simulink model "PMSM_Model_fixed"  (R2022b)
settings: Solver=ode23t  StartTime=0.0  StopTime=0.5  RelTol=1e-3
model workspace (MAT data in the model file):
  Ki = 1000
  Kp = 2
  Ts_ctrl = 0.0001
  Ts_norm = 1
  Vdc = 100
  fsw = 10000
  p = 6
undefined symbols (not defined in the file): docblock
libraries: nesl_utility x11, fl_lib x10, ee_lib x4, spsTriangleGeneratorLib x1
settings Model: Creator=59263  LastModifiedBy=59263

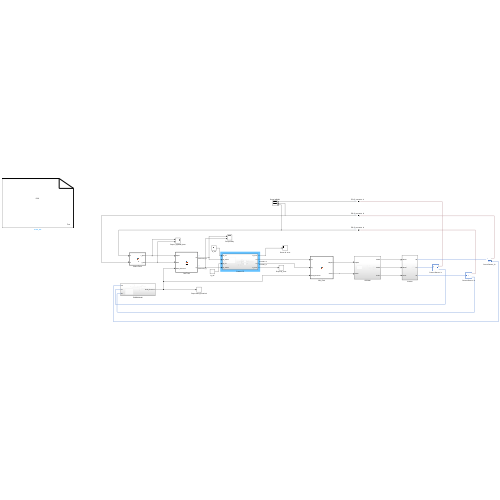
[thumbnail: Simulink's stored preview of the top-level diagram]
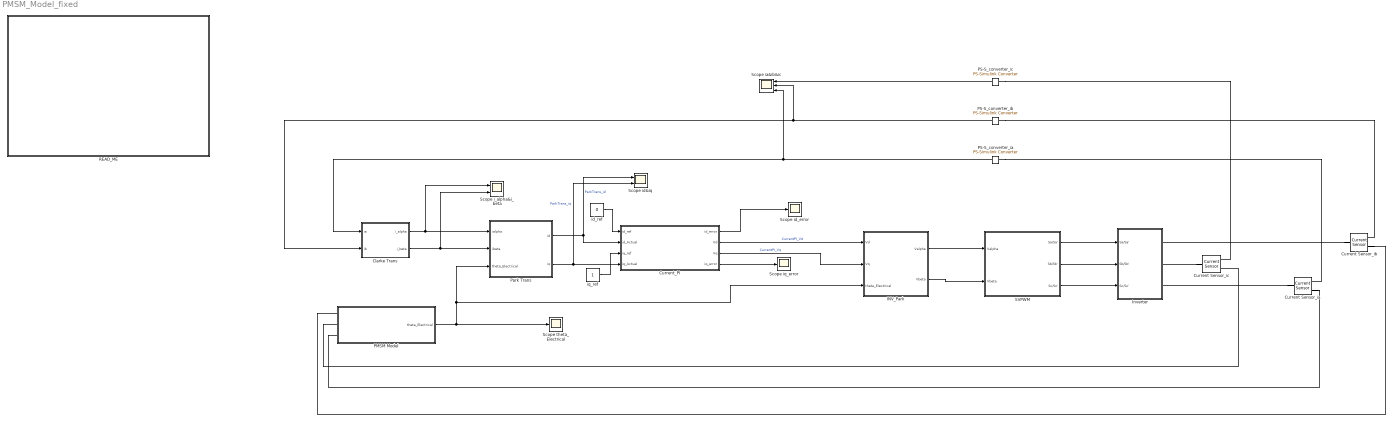
== system PMSM_Model_fixed ==
  Clarke Trans : MATLAB Function  TreatAsAtomicUnit=on
  Current Sensor_ia : fl_lib/Electrical/Electrical Sensors/Current Sensor
  Current Sensor_ib : fl_lib/Electrical/Electrical Sensors/Current Sensor
  Current Sensor_ic : fl_lib/Electrical/Electrical Sensors/Current Sensor
  Current_PI : Subsystem
  INV_Park : MATLAB Function  TreatAsAtomicUnit=on
  Inverter : Subsystem
  PMSM Model : Subsystem
  PS-S_converter_ia : nesl_utility/PS-Simulink Converter  PhysicalDomain=network_engine_domain  SubClassName=ps_output  LeftPortType=input  RightPortType=output  PseudoPeriodic=off  Frequencies=[]  VectorFormat=inherit  Unit=A  AffineConversion=off
  PS-S_converter_ib : nesl_utility/PS-Simulink Converter  PhysicalDomain=network_engine_domain  SubClassName=ps_output  LeftPortType=input  RightPortType=output  PseudoPeriodic=off  Frequencies=[]  VectorFormat=inherit  Unit=A  AffineConversion=off
  PS-S_converter_ic : nesl_utility/PS-Simulink Converter  PhysicalDomain=network_engine_domain  SubClassName=ps_output  LeftPortType=input  RightPortType=output  PseudoPeriodic=off  Frequencies=[]  VectorFormat=inherit  Unit=inherit  AffineConversion=off
  Park Trans : MATLAB Function  TreatAsAtomicUnit=on
  READ_ME : Subsystem  InitFcn=docblock('save_document',gcb);  mask(DocBlock){ECoderFlag=, DocumentType=Text}
      mask prompts: ECoderFlag "Simulink:masks:DocBlockEmbeddedCoderFlagLabel_MP"; DocumentType "Simulink:masks:DocBlockDocTypeLabel_MP"
      mask help:
      | PMSM 矢量控制（FOC）仿真模型 —— 表贴式 PMSM，i_d* = 0，i_q* = 1 A
      |
      | 【功能分层】
      |   Inverter     三相两电平电压源逆变器（3 x Half-Bridge）+ 直流母线 + 电压传感
      |   PMSM Model   PMSM 本体 + 旋转传感器 + 位置处理，输出电角度 theta_Electrical
      |   Current_PI   dq 电流环（离散 PI + 一拍计算延迟），输出 Vd / Vq 及 id/iq 误差
      |   SVPWM        空间矢量调制：abc_PWM（扇区/T1T2/占空比）+ 载波比较 + 互补门极
      |
      | 【模型工作区变量】改参数请改这里，不要钻进子系统改
      |   Kp      = 2      电流环比例增益
      |   Ki      = 1000   电流环积分增益（Ki/Kp = R/L = 500，Kp = wc*L）
      |   Vdc     = 100    直流母线电压 [V]（同时驱动 DC 源、SVPWM 的 Vdc）
      |   Ts_norm = 1      SVPWM 归一化周期（Ts=1 时 Da/Db/Dc 直接就是占空比）
      |   Ts_ctrl = 1e-4   电流环采样周期 [s]，10 kHz，与载波同频
      |   fsw     = 1e4    三角载波频率 [Hz]
      |   p       = 6      极对数（同时驱动 PMSM 本体和 theta 换算的 Gain）
      |
      | 【运行】StopTime = 0.5 s，变步长 ode23t，RelTol = 1e-3
      |
      | 【改参数时的联动关系】
      |   Vdc  ->  同时影响 DC 源、SVPWM 占空比计算
      |         ->  PI 脚本里硬编码的限幅 limit = 57 V (= Vdc/sqrt(3)) 也要同步改
      |   Ts_ctrl/p/fsw -> 见 Current_PI 与 SVPWM 子系统里的说明
      settings: DeleteFcn=docblock('close_document',gcb);  PreSaveFcn=docblock('save_document',gcb);  OpenFcn=docblock('edit_document',gcb);
      settings: LibrarySourceBlock=|
      | simulink/Model-Wide
      | Utilities/DocBlock
      mask TypeOptions DocumentType: Simulink:masks:Text | Simulink:masks:RTF | Simulink:masks:HTML
      mask Display:
      | plot([.8 0 0 1 1 .8 .8 1],[1 1 0 0 .8 1 .8 .8]);
      | text(.5,.6,'DOC','horizontalalignment','center');
      | text(.95,.05,get_param(gcb,'DocumentType'),'verticalalignment','bottom','horizontalalignment','right');
  SVPWM : Subsystem
  Scope i_alpha&i_beta : Scope  NumInputPorts=2
  Scope ia&ib&ic : Scope  NumInputPorts=3
  Scope id&iq : Scope  NumInputPorts=2
  Scope id_error : Scope
  Scope iq_error : Scope
  Scope theta_Electrical : Scope
  id_ref : Constant  Value=0
  iq_ref : Constant
  wires:
  PS-S_converter_ia/1 -> Clarke Trans/1(ia), Scope ia&ib&ic/3
  PS-S_converter_ib/1 -> Clarke Trans/2(ib), Scope ia&ib&ic/2
  Clarke Trans/1(i_alpha) -> Scope i_alpha&i_beta/1, Park Trans/1(ialpha)
  Clarke Trans/2(i_beta) -> Scope i_alpha&i_beta/2, Park Trans/2(ibeta)
  Park Trans/1(id) -> Current_PI/2(id_Actual), Scope id&iq/1  "ParkTrans_id"
  Park Trans/2(iq) -> Current_PI/4(iq_Actual), Scope id&iq/2  "ParkTrans_iq"
  INV_Park/1(Valpha) -> SVPWM/1(Valpha)
  INV_Park/2(Vbeta) -> SVPWM/2(Vbeta)
  SVPWM/1(Sa/Sa') -> Inverter/1(Sa/Sa')
  SVPWM/2(Sb/Sb') -> Inverter/2(Sb/Sb')
  SVPWM/3(Sc/Sc') -> Inverter/3(Sc/Sc')
  Current_PI/1(id_error) -> Scope id_error/1
  Current_PI/2(Vd) -> INV_Park/1(Vd)  "CurrentPI_Vd"
  Current_PI/3(Vq) -> INV_Park/2(Vq)  "CurrentPI_Vq"
  Current_PI/4(iq_error) -> Scope iq_error/1
  PMSM Model/1(theta_Electrical) -> Scope theta_Electrical/1, Park Trans/3(theta_Electrical), INV_Park/3(theta_Electrical)
  PS-S_converter_ic/1 -> Scope ia&ib&ic/1
  id_ref/1 -> Current_PI/1(id_ref)
  iq_ref/1 -> Current_PI/3(iq_ref)
  connections:
  PS-S_converter_ia/LConn1 -- Current Sensor_ia/RConn1
  PS-S_converter_ib/LConn1 -- Current Sensor_ib/RConn1
  PS-S_converter_ic/LConn1 -- Current Sensor_ic/RConn1
  Current Sensor_ib/LConn1 -- Inverter/RConn1
  Current Sensor_ic/LConn1 -- Inverter/RConn2
  Current Sensor_ia/LConn1 -- Inverter/RConn3
  Current Sensor_ib/RConn2 -- PMSM Model/LConn1
  PMSM Model/LConn2 -- Current Sensor_ic/RConn2
  Current Sensor_ia/RConn2 -- PMSM Model/LConn3

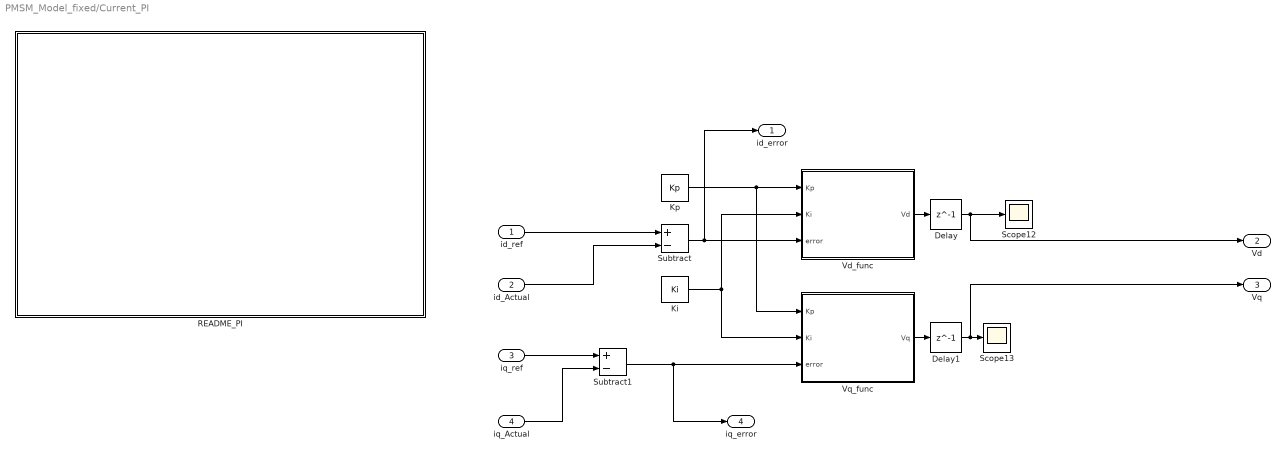
== system PMSM_Model_fixed/Current_PI ==
  id_ref : Inport
  id_Actual : Inport  Port=2
  iq_ref : Inport  Port=3
  iq_Actual : Inport  Port=4
  Delay : Delay  DelayLength=1  SampleTime=Ts_ctrl
  Delay1 : Delay  DelayLength=1  SampleTime=Ts_ctrl
  Ki : Constant  Value=Ki
  Kp : Constant  Value=Kp
  README_PI : Subsystem  InitFcn=docblock('save_document',gcb);  mask(DocBlock){ECoderFlag=, DocumentType=Text}
      mask prompts: ECoderFlag "Simulink:masks:DocBlockEmbeddedCoderFlagLabel_MP"; DocumentType "Simulink:masks:DocBlockDocTypeLabel_MP"
      mask help:
      | dq 轴电流环（离散 PI）
      |
      | 【接口】
      |   输入：id_ref、id_Actual、iq_ref、iq_Actual
      |   输出：id_error、Vd、Vq、iq_error
      |
      | 【结构】
      |   Subtract(+-)  -> id_error -> Vd_func -> Delay (Ts_ctrl) -> Vd
      |   Subtract1(+-) -> iq_error -> Vq_func -> Delay1(Ts_ctrl) -> Vq
      |
      | 【增益】Kp / Ki 引用模型工作区变量（默认 2 / 1000）
      |   整定依据：对象 1/(Ls+R)，L = 1 mH，R = 0.5 ohm
      |     零极点对消：Ki/Kp = R/L = 500
      |     穿越频率  ：wc = Kp/L = 2000 rad/s ≈ 318 Hz（约 fsw/31）
      |     相位裕度  ：PM ≈ 90 - wc*Td ≈ 67 度（Td ≈ 2 个采样周期）
      |
      | 【!! 采样时间一致性 !!】
      |   两个 PI 图表必须保持 ChartUpdate = DISCRETE、SampleTime = 1e-4，
      |   并且脚本里的字面量 Ts 必须等于该采样时间。
      |   若图表是 INHERITED（连续），在变步长求解器下积分量会被重复累加
      |   约两个数量级，整定参数完全失效 —— 这是最难查的一类静默错误。
      |
      | 【限幅】Vd / Vq 的限幅 ±57 V 硬编码在脚本里 = Vdc/sqrt(3)，改 Vdc 时要同步改。
      settings: DeleteFcn=docblock('close_document',gcb);  PreSaveFcn=docblock('save_document',gcb);  OpenFcn=docblock('edit_document',gcb);
      settings: LibrarySourceBlock=|
      | simulink/Model-Wide
      | Utilities/DocBlock
      mask TypeOptions DocumentType: Simulink:masks:Text | Simulink:masks:RTF | Simulink:masks:HTML
      mask Display:
      | plot([.8 0 0 1 1 .8 .8 1],[1 1 0 0 .8 1 .8 .8]);
      | text(.5,.6,'DOC','horizontalalignment','center');
      | text(.95,.05,get_param(gcb,'DocumentType'),'verticalalignment','bottom','horizontalalignment','right');
  Scope12 : Scope
  Scope13 : Scope
  Subtract : Sum  Inputs=+-
  Subtract1 : Sum  Inputs=+-
  Vd_func : MATLAB Function  TreatAsAtomicUnit=on
  Vq_func : MATLAB Function  TreatAsAtomicUnit=on
  id_error : Outport
  Vd : Outport  Port=2
  Vq : Outport  Port=3
  iq_error : Outport  Port=4
  wires:
  Vd_func/1(Vd) -> Delay/1
  Delay/1 -> Vd/1, Scope12/1
  Subtract/1 -> id_error/1, Vd_func/3(error)
  Vq_func/1(Vq) -> Delay1/1
  id_ref/1 -> Subtract/1
  Delay1/1 -> Vq/1, Scope13/1
  Ki/1 -> Vq_func/2(Ki), Vd_func/2(Ki)
  Subtract1/1 -> Vq_func/3(error), iq_error/1
  id_Actual/1 -> Subtract/2
  Kp/1 -> Vd_func/1(Kp), Vq_func/1(Kp)
  iq_ref/1 -> Subtract1/1
  iq_Actual/1 -> Subtract1/2

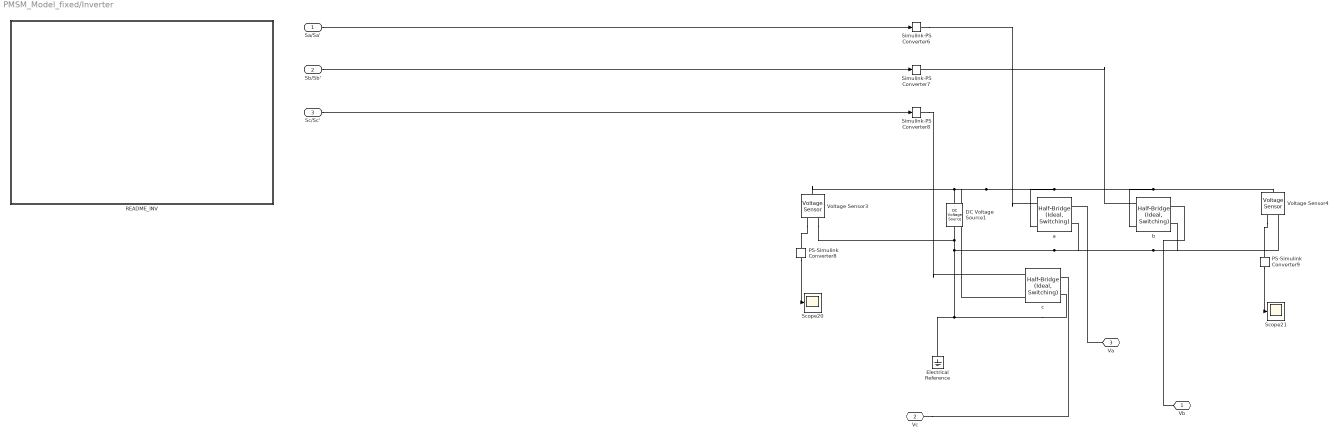
== system PMSM_Model_fixed/Inverter ==
  Sa/Sa' : Inport
  Sb/Sb' : Inport  Port=2
  Sc/Sc' : Inport  Port=3
  DC Voltage Source1 : fl_lib/Electrical/Electrical Sources/DC Voltage Source  v0=Vdc V
  Electrical Reference : fl_lib/Electrical/Electrical Elements/Electrical Reference
  PS-Simulink Converter8 : nesl_utility/PS-Simulink Converter  PhysicalDomain=network_engine_domain  SubClassName=ps_output  LeftPortType=input  RightPortType=output  PseudoPeriodic=off  Frequencies=[]  VectorFormat=inherit  Unit=inherit  AffineConversion=off
  PS-Simulink Converter9 : nesl_utility/PS-Simulink Converter  PhysicalDomain=network_engine_domain  SubClassName=ps_output  LeftPortType=input  RightPortType=output  PseudoPeriodic=off  Frequencies=[]  VectorFormat=inherit  Unit=inherit  AffineConversion=off
  README_INV : Subsystem  InitFcn=docblock('save_document',gcb);  mask(DocBlock){ECoderFlag=, DocumentType=Text}
      mask prompts: ECoderFlag "Simulink:masks:DocBlockEmbeddedCoderFlagLabel_MP"; DocumentType "Simulink:masks:DocBlockDocTypeLabel_MP"
      mask help:
      | 三相两电平电压源型逆变器
      |
      | 【接口】
      |   信号输入 Sa/Sa'、Sb/Sb'、Sc/Sc'：每路 2 元素向量 [上管门极, 下管门极]，互补
      |   物理端口 Va / Vb / Vc（块上顺序是 Vb / Vc / Va）：三个桥臂中点
      |
      | 【器件设置】
      |   device_type = MOSFET (Ideal, Switching)，mosfet_Vth = 0.5 V
      |   ! 阈值必须匹配门极信号电平（0/1 逻辑 -> 0.5 V）。
      |     若换成 GTO，阈值变成 gto_Vgt = 6 V，0/1 信号将无法开通。
      |   ! diode_param = include.no：半桥不含反并联续流二极管，
      |     因此必须用互补门极提供续流通路（已由 SVPWM 侧的 NOT + Mux 保证）。
      |     真实逆变器一定有体二极管或反并联二极管。
      |
      | 【其他】
      |   DC Voltage Source1 的 v0 = Vdc（模型工作区变量）
      |   Voltage Sensor3/4 跨接在直流母线上，测的是母线电压（冗余，控制未使用）
      settings: DeleteFcn=docblock('close_document',gcb);  PreSaveFcn=docblock('save_document',gcb);  OpenFcn=docblock('edit_document',gcb);
      settings: LibrarySourceBlock=|
      | simulink/Model-Wide
      | Utilities/DocBlock
      mask TypeOptions DocumentType: Simulink:masks:Text | Simulink:masks:RTF | Simulink:masks:HTML
      mask Display:
      | plot([.8 0 0 1 1 .8 .8 1],[1 1 0 0 .8 1 .8 .8]);
      | text(.5,.6,'DOC','horizontalalignment','center');
      | text(.95,.05,get_param(gcb,'DocumentType'),'verticalalignment','bottom','horizontalalignment','right');
  Scope20 : Scope
  Scope21 : Scope
  Simulink-PS Converter6 : nesl_utility/Simulink-PS Converter  PhysicalDomain=network_engine_domain  SubClassName=ps_input  LeftPortType=input  RightPortType=output  PseudoPeriodic=off  Frequencies=[]  NoiseDistribution=none  NoiseParameters=[]  Unit=1  AffineConversion=off  FilteringAndDerivatives=provide  SimscapeFilterOrder=1  InputFilterTimeConstant=0.001  UdotUserProvided=0
  Simulink-PS Converter7 : nesl_utility/Simulink-PS Converter  PhysicalDomain=network_engine_domain  SubClassName=ps_input  LeftPortType=input  RightPortType=output  PseudoPeriodic=off  Frequencies=[]  NoiseDistribution=none  NoiseParameters=[]  Unit=1  AffineConversion=off  FilteringAndDerivatives=provide  SimscapeFilterOrder=1  InputFilterTimeConstant=0.001  UdotUserProvided=0
  Simulink-PS Converter8 : nesl_utility/Simulink-PS Converter  PhysicalDomain=network_engine_domain  SubClassName=ps_input  LeftPortType=input  RightPortType=output  PseudoPeriodic=off  Frequencies=[]  NoiseDistribution=none  NoiseParameters=[]  Unit=1  AffineConversion=off  FilteringAndDerivatives=provide  SimscapeFilterOrder=1  InputFilterTimeConstant=0.001  UdotUserProvided=0
  Voltage Sensor3 : fl_lib/Electrical/Electrical Sensors/Voltage Sensor
  Voltage Sensor4 : fl_lib/Electrical/Electrical Sensors/Voltage Sensor
  a : ee_lib/Semiconductors & Converters/Half-Bridge (Ideal, Switching)  control_port=ee.enum.controlport.ps  device_type=ee.enum.converters.switches.mosfet  gto_Vgt=6 V  gto_Vgt_off=-1 V  gto_Ih=1 A  gto_thermal_loss_option=ee.enum.converters.thermalLossOption.constantvalues  gto_Vf=0.8 V  gto_Ron=0.001 Ohm  gto_Von_data=[0, .1, .6, .8, 1, 1.3, 1.6, 2, 2.4; 0, .1, .7, 1, 1.2, 1.5, 1.9, 2.4, 2.8] V  gto_Tj=[298.15, 398.15] K  gto_Iout_data=[0, .1, 1, 5, 10, 20, 40, 70, 100] A  igbt_Vth=6 V  igbt_thermal_loss_option=ee.enum.converters.thermalLossOption.constantvalues  igbt_Vf=0.8 V  igbt_Ron=0.001 Ohm  igbt_Von_data=[0, .1, .6, .8, 1, 1.3, 1.6, 2, 2.4; 0, .1, .7, 1, 1.2, 1.5, 1.9, 2.4, 2.8] V  igbt_Tj=[298.15, 398.15] K  igbt_Iout_data=[0, .1, 1, 5, 10, 20, 40, 70, 100] A  mosfet_Vth=0.5 V  mosfet_thermal_loss_option=ee.enum.converters.thermalLossOption.constantvalues  mosfet_Rds=0.01 Ohm  mosfet_Von_data=[0, 1.1, 1.3, 1.45, 1.75, 2.25, 2.7; 0, 1, 1.15, 1.35, 1.7, 2.35, 3] V  mosfet_Tj=[298.15, 398.15] K  mosfet_Iout_data=[0, 10, 50, 100, 200, 400, 600] A  Goff=1e-6 1/Ohm  gto_Eon_data=[0, .0024, .024, .12, .2, .48, 1.04, 2.16, 3.24; 0, .003, .03, .15, .25, .6, 1.3, 2.7, 4.05] * 1e-3 J  gto_Eoff_data=[0, .0007, .0066, .033, .066, .17, .33, .83, 1.5; 0, .001, .01, .05, .1, .25, .5, 1.2, 2.2] * 1e-3 J  gto_Erec_data=[0, .0031, .021, .11, .21, .43, .99, 1.71, 3.078; 0, .0041, .043, .2, .39, .77, 1.54, 2.27, 4.08] * 1e-3 J  gto_Tj_loss=[298.15, 398.15] K  gto_Iout_data_loss=[0, .1, 1, 5, 10, 20, 40, 70, 100] A  gto_Eon_scalar=22.86e-3 J  gto_Eoff_scalar=17.14e-3 J  gto_Eoff_natural_commutation=10e-3 J  gto_Erec_scalar=5.70e-3 J  gto_Iout_scalar=600 A  igbt_Eon_data=[0, .0024, .024, .12, .2, .48, 1.04, 2.16, 3.24; 0, .003, .03, .15, .25, .6, 1.3, 2.7, 4.05] * 1e-3 J  igbt_Eoff_data=[0, .0007, .0066, .033, .066, .17, .33, .83, 1.5; 0, .001, .01, .05, .1, .25, .5, 1.2, 2.2] * 1e-3 J  igbt_Erec_data=[0, .0031, .021, .11, .21, .43, .99, 1.71, 3.078; 0, .0041, .043, .2, .39, .77, 1.54, 2.27, 4.08] * 1e-3 J  igbt_Tj_loss=[298.15, 398.15] K  igbt_Iout_data_loss=[0, .1, 1, 5, 10, 20, 40, 70, 100] A  igbt_Eon_scalar=22.86e-3 J  igbt_Eoff_scalar=17.14e-3 J  igbt_Erec_scalar=5.70e-3 J  igbt_Iout_scalar=600 A  mosfet_Eon_data=[0, .29, 1.43, 2.86, 5.71, 13.14, 22.86; 0, .57, 2.63, 5.14, 10.29, 20.57, 30.29] * 1e-3 J  mosfet_Eoff_data=[0, .21, 1.07, 2.14, 4.29, 9.86, 17.14; 0, .43, 1.97, 3.86, 7.71, 15.43, 22.71] * 1e-3 J  mosfet_Erec_data=[0, .0031, .021, .11, .21, .43, .99, 1.71, 3.078; 0, .0041, .043, .2, .39, .77, 1.54, 2.27, 4.08] * 1e-3 J  mosfet_Tj_loss=[298.15, 398.15] K  mosfet_Iout_data_loss=[0, 10, 50, 100, 200, 400, 600] A  mosfet_Eon_scalar=22.86e-3 J  mosfet_Eoff_scalar=17.14e-3 J  mosfet_Erec_scalar=5.70e-3 J  mosfet_Iout_scalar=600 A  Voff=300 V  diode_param=ee.enum.include.no  diode_ModelType=ee.enum.converters.diodeModelType.pwl  diode_TableType=ee.enum.diode.tableType.IfMat  diode_IfMat=[.07, .12, .19, 1.75, 4.24, 7.32, 11.2; .16, .3, .72, 2.14, 4.02, 6.35, 9.12] A  diode_VfMat=[.9, 1.15, 1.25, 1.5, 1.75, 2.17, 2.6, 2.85; .58, .68, .75, 1.1, 1.38, 1.77, 2.27, 2.7] V  diode_TjVec=[25, 125] degC  diode_VfVec=[.5, .7, .9, 1.3, 1.7, 2.1, 2.5] V  diode_IfVec=[.1, .2, .5, 1, 2, 4, 7, 10] A  diode_Vf=0.8 V  diode_Ron=0.001 Ohm  diode_Goff=1e-5 1/Ohm  thermal_network_parameterization=ee.enum.thermalNetworkTopology.external  Rth=[.03, .2] K/W  Rth_Cauer=[.03, .1, .2] K/W  Rth_Foster=[.03, .2] K/W  thermal_mass_parameterization=ee.enum.thermalNetwork.timeconstant  thermal_mass=[3, 25] J/K  thermal_mass_Cauer=[3, 10, 25] J/K  thermal_mass_Foster=[33, 50] J/K  thermal_time_constant=[.1, 5] s  thermal_time_constant_Cauer=[.1, 1, 5] s  thermal_time_constant_Foster=[1, 10] s  thermal_mass_initial_temperatures=[25, 25] degC  thermal_mass_initial_temperatures_Cauer=[25, 25, 25] degC  junction_thermal_mass=0.1 J/K  Tvec_initial_Foster=[25, 25, 25, 25] degC  junction_temperature_specify=off  junction_temperature_priority=None  junction_temperature=25 degC  junction_temperature_nominal_specify=off  junction_temperature_nominal_unit=degC  junction_temperature_nominal_value=1
      settings: InternalSimscapePortConfiguration="{\"Bottom\":[{\"id\":\"n\",\"label\":\"-\",\"type\":\"foundation.electrical.electrical\"}],\"Left\":[{\"id\":\"G\",\"label\":\"G\",\"type\":\"input\"},{\"id\":\"H\",\"label\":\"\",\"type\":\"foundation.thermal.thermal\"}],\"Right\":[{\"id\":\"o\",\"label\":\"o\",\"type\":\"foundation.electrical.electrical\"}],\"Top\":[{\"id\":\"p\",\"label\":\"+\",\"type\":\"foundation.electrical.electrical\"}]}"
  b : ee_lib/Semiconductors & Converters/Half-Bridge (Ideal, Switching)  control_port=ee.enum.controlport.ps  device_type=ee.enum.converters.switches.mosfet  gto_Vgt=6 V  gto_Vgt_off=-1 V  gto_Ih=1 A  gto_thermal_loss_option=ee.enum.converters.thermalLossOption.constantvalues  gto_Vf=0.8 V  gto_Ron=0.001 Ohm  gto_Von_data=[0, .1, .6, .8, 1, 1.3, 1.6, 2, 2.4; 0, .1, .7, 1, 1.2, 1.5, 1.9, 2.4, 2.8] V  gto_Tj=[298.15, 398.15] K  gto_Iout_data=[0, .1, 1, 5, 10, 20, 40, 70, 100] A  igbt_Vth=6 V  igbt_thermal_loss_option=ee.enum.converters.thermalLossOption.constantvalues  igbt_Vf=0.8 V  igbt_Ron=0.001 Ohm  igbt_Von_data=[0, .1, .6, .8, 1, 1.3, 1.6, 2, 2.4; 0, .1, .7, 1, 1.2, 1.5, 1.9, 2.4, 2.8] V  igbt_Tj=[298.15, 398.15] K  igbt_Iout_data=[0, .1, 1, 5, 10, 20, 40, 70, 100] A  mosfet_Vth=0.5 V  mosfet_thermal_loss_option=ee.enum.converters.thermalLossOption.constantvalues  mosfet_Rds=0.01 Ohm  mosfet_Von_data=[0, 1.1, 1.3, 1.45, 1.75, 2.25, 2.7; 0, 1, 1.15, 1.35, 1.7, 2.35, 3] V  mosfet_Tj=[298.15, 398.15] K  mosfet_Iout_data=[0, 10, 50, 100, 200, 400, 600] A  Goff=1e-6 1/Ohm  gto_Eon_data=[0, .0024, .024, .12, .2, .48, 1.04, 2.16, 3.24; 0, .003, .03, .15, .25, .6, 1.3, 2.7, 4.05] * 1e-3 J  gto_Eoff_data=[0, .0007, .0066, .033, .066, .17, .33, .83, 1.5; 0, .001, .01, .05, .1, .25, .5, 1.2, 2.2] * 1e-3 J  gto_Erec_data=[0, .0031, .021, .11, .21, .43, .99, 1.71, 3.078; 0, .0041, .043, .2, .39, .77, 1.54, 2.27, 4.08] * 1e-3 J  gto_Tj_loss=[298.15, 398.15] K  gto_Iout_data_loss=[0, .1, 1, 5, 10, 20, 40, 70, 100] A  gto_Eon_scalar=22.86e-3 J  gto_Eoff_scalar=17.14e-3 J  gto_Eoff_natural_commutation=10e-3 J  gto_Erec_scalar=5.70e-3 J  gto_Iout_scalar=600 A  igbt_Eon_data=[0, .0024, .024, .12, .2, .48, 1.04, 2.16, 3.24; 0, .003, .03, .15, .25, .6, 1.3, 2.7, 4.05] * 1e-3 J  igbt_Eoff_data=[0, .0007, .0066, .033, .066, .17, .33, .83, 1.5; 0, .001, .01, .05, .1, .25, .5, 1.2, 2.2] * 1e-3 J  igbt_Erec_data=[0, .0031, .021, .11, .21, .43, .99, 1.71, 3.078; 0, .0041, .043, .2, .39, .77, 1.54, 2.27, 4.08] * 1e-3 J  igbt_Tj_loss=[298.15, 398.15] K  igbt_Iout_data_loss=[0, .1, 1, 5, 10, 20, 40, 70, 100] A  igbt_Eon_scalar=22.86e-3 J  igbt_Eoff_scalar=17.14e-3 J  igbt_Erec_scalar=5.70e-3 J  igbt_Iout_scalar=600 A  mosfet_Eon_data=[0, .29, 1.43, 2.86, 5.71, 13.14, 22.86; 0, .57, 2.63, 5.14, 10.29, 20.57, 30.29] * 1e-3 J  mosfet_Eoff_data=[0, .21, 1.07, 2.14, 4.29, 9.86, 17.14; 0, .43, 1.97, 3.86, 7.71, 15.43, 22.71] * 1e-3 J  mosfet_Erec_data=[0, .0031, .021, .11, .21, .43, .99, 1.71, 3.078; 0, .0041, .043, .2, .39, .77, 1.54, 2.27, 4.08] * 1e-3 J  mosfet_Tj_loss=[298.15, 398.15] K  mosfet_Iout_data_loss=[0, 10, 50, 100, 200, 400, 600] A  mosfet_Eon_scalar=22.86e-3 J  mosfet_Eoff_scalar=17.14e-3 J  mosfet_Erec_scalar=5.70e-3 J  mosfet_Iout_scalar=600 A  Voff=300 V  diode_param=ee.enum.include.no  diode_ModelType=ee.enum.converters.diodeModelType.pwl  diode_TableType=ee.enum.diode.tableType.IfMat  diode_IfMat=[.07, .12, .19, 1.75, 4.24, 7.32, 11.2; .16, .3, .72, 2.14, 4.02, 6.35, 9.12] A  diode_VfMat=[.9, 1.15, 1.25, 1.5, 1.75, 2.17, 2.6, 2.85; .58, .68, .75, 1.1, 1.38, 1.77, 2.27, 2.7] V  diode_TjVec=[25, 125] degC  diode_VfVec=[.5, .7, .9, 1.3, 1.7, 2.1, 2.5] V  diode_IfVec=[.1, .2, .5, 1, 2, 4, 7, 10] A  diode_Vf=0.8 V  diode_Ron=0.001 Ohm  diode_Goff=1e-5 1/Ohm  thermal_network_parameterization=ee.enum.thermalNetworkTopology.external  Rth=[.03, .2] K/W  Rth_Cauer=[.03, .1, .2] K/W  Rth_Foster=[.03, .2] K/W  thermal_mass_parameterization=ee.enum.thermalNetwork.timeconstant  thermal_mass=[3, 25] J/K  thermal_mass_Cauer=[3, 10, 25] J/K  thermal_mass_Foster=[33, 50] J/K  thermal_time_constant=[.1, 5] s  thermal_time_constant_Cauer=[.1, 1, 5] s  thermal_time_constant_Foster=[1, 10] s  thermal_mass_initial_temperatures=[25, 25] degC  thermal_mass_initial_temperatures_Cauer=[25, 25, 25] degC  junction_thermal_mass=0.1 J/K  Tvec_initial_Foster=[25, 25, 25, 25] degC  junction_temperature_specify=off  junction_temperature_priority=None  junction_temperature=25 degC  junction_temperature_nominal_specify=off  junction_temperature_nominal_unit=degC  junction_temperature_nominal_value=1
      settings: InternalSimscapePortConfiguration="{\"Bottom\":[{\"id\":\"n\",\"label\":\"-\",\"type\":\"foundation.electrical.electrical\"}],\"Left\":[{\"id\":\"G\",\"label\":\"G\",\"type\":\"input\"},{\"id\":\"H\",\"label\":\"\",\"type\":\"foundation.thermal.thermal\"}],\"Right\":[{\"id\":\"o\",\"label\":\"o\",\"type\":\"foundation.electrical.electrical\"}],\"Top\":[{\"id\":\"p\",\"label\":\"+\",\"type\":\"foundation.electrical.electrical\"}]}"
  c : ee_lib/Semiconductors & Converters/Half-Bridge (Ideal, Switching)  control_port=ee.enum.controlport.ps  device_type=ee.enum.converters.switches.mosfet  gto_Vgt=6 V  gto_Vgt_off=-1 V  gto_Ih=1 A  gto_thermal_loss_option=ee.enum.converters.thermalLossOption.constantvalues  gto_Vf=0.8 V  gto_Ron=0.001 Ohm  gto_Von_data=[0, .1, .6, .8, 1, 1.3, 1.6, 2, 2.4; 0, .1, .7, 1, 1.2, 1.5, 1.9, 2.4, 2.8] V  gto_Tj=[298.15, 398.15] K  gto_Iout_data=[0, .1, 1, 5, 10, 20, 40, 70, 100] A  igbt_Vth=6 V  igbt_thermal_loss_option=ee.enum.converters.thermalLossOption.constantvalues  igbt_Vf=0.8 V  igbt_Ron=0.001 Ohm  igbt_Von_data=[0, .1, .6, .8, 1, 1.3, 1.6, 2, 2.4; 0, .1, .7, 1, 1.2, 1.5, 1.9, 2.4, 2.8] V  igbt_Tj=[298.15, 398.15] K  igbt_Iout_data=[0, .1, 1, 5, 10, 20, 40, 70, 100] A  mosfet_Vth=0.5 V  mosfet_thermal_loss_option=ee.enum.converters.thermalLossOption.constantvalues  mosfet_Rds=0.01 Ohm  mosfet_Von_data=[0, 1.1, 1.3, 1.45, 1.75, 2.25, 2.7; 0, 1, 1.15, 1.35, 1.7, 2.35, 3] V  mosfet_Tj=[298.15, 398.15] K  mosfet_Iout_data=[0, 10, 50, 100, 200, 400, 600] A  Goff=1e-6 1/Ohm  gto_Eon_data=[0, .0024, .024, .12, .2, .48, 1.04, 2.16, 3.24; 0, .003, .03, .15, .25, .6, 1.3, 2.7, 4.05] * 1e-3 J  gto_Eoff_data=[0, .0007, .0066, .033, .066, .17, .33, .83, 1.5; 0, .001, .01, .05, .1, .25, .5, 1.2, 2.2] * 1e-3 J  gto_Erec_data=[0, .0031, .021, .11, .21, .43, .99, 1.71, 3.078; 0, .0041, .043, .2, .39, .77, 1.54, 2.27, 4.08] * 1e-3 J  gto_Tj_loss=[298.15, 398.15] K  gto_Iout_data_loss=[0, .1, 1, 5, 10, 20, 40, 70, 100] A  gto_Eon_scalar=22.86e-3 J  gto_Eoff_scalar=17.14e-3 J  gto_Eoff_natural_commutation=10e-3 J  gto_Erec_scalar=5.70e-3 J  gto_Iout_scalar=600 A  igbt_Eon_data=[0, .0024, .024, .12, .2, .48, 1.04, 2.16, 3.24; 0, .003, .03, .15, .25, .6, 1.3, 2.7, 4.05] * 1e-3 J  igbt_Eoff_data=[0, .0007, .0066, .033, .066, .17, .33, .83, 1.5; 0, .001, .01, .05, .1, .25, .5, 1.2, 2.2] * 1e-3 J  igbt_Erec_data=[0, .0031, .021, .11, .21, .43, .99, 1.71, 3.078; 0, .0041, .043, .2, .39, .77, 1.54, 2.27, 4.08] * 1e-3 J  igbt_Tj_loss=[298.15, 398.15] K  igbt_Iout_data_loss=[0, .1, 1, 5, 10, 20, 40, 70, 100] A  igbt_Eon_scalar=22.86e-3 J  igbt_Eoff_scalar=17.14e-3 J  igbt_Erec_scalar=5.70e-3 J  igbt_Iout_scalar=600 A  mosfet_Eon_data=[0, .29, 1.43, 2.86, 5.71, 13.14, 22.86; 0, .57, 2.63, 5.14, 10.29, 20.57, 30.29] * 1e-3 J  mosfet_Eoff_data=[0, .21, 1.07, 2.14, 4.29, 9.86, 17.14; 0, .43, 1.97, 3.86, 7.71, 15.43, 22.71] * 1e-3 J  mosfet_Erec_data=[0, .0031, .021, .11, .21, .43, .99, 1.71, 3.078; 0, .0041, .043, .2, .39, .77, 1.54, 2.27, 4.08] * 1e-3 J  mosfet_Tj_loss=[298.15, 398.15] K  mosfet_Iout_data_loss=[0, 10, 50, 100, 200, 400, 600] A  mosfet_Eon_scalar=22.86e-3 J  mosfet_Eoff_scalar=17.14e-3 J  mosfet_Erec_scalar=5.70e-3 J  mosfet_Iout_scalar=600 A  Voff=300 V  diode_param=ee.enum.include.no  diode_ModelType=ee.enum.converters.diodeModelType.pwl  diode_TableType=ee.enum.diode.tableType.IfMat  diode_IfMat=[.07, .12, .19, 1.75, 4.24, 7.32, 11.2; .16, .3, .72, 2.14, 4.02, 6.35, 9.12] A  diode_VfMat=[.9, 1.15, 1.25, 1.5, 1.75, 2.17, 2.6, 2.85; .58, .68, .75, 1.1, 1.38, 1.77, 2.27, 2.7] V  diode_TjVec=[25, 125] degC  diode_VfVec=[.5, .7, .9, 1.3, 1.7, 2.1, 2.5] V  diode_IfVec=[.1, .2, .5, 1, 2, 4, 7, 10] A  diode_Vf=0.8 V  diode_Ron=0.001 Ohm  diode_Goff=1e-5 1/Ohm  thermal_network_parameterization=ee.enum.thermalNetworkTopology.external  Rth=[.03, .2] K/W  Rth_Cauer=[.03, .1, .2] K/W  Rth_Foster=[.03, .2] K/W  thermal_mass_parameterization=ee.enum.thermalNetwork.timeconstant  thermal_mass=[3, 25] J/K  thermal_mass_Cauer=[3, 10, 25] J/K  thermal_mass_Foster=[33, 50] J/K  thermal_time_constant=[.1, 5] s  thermal_time_constant_Cauer=[.1, 1, 5] s  thermal_time_constant_Foster=[1, 10] s  thermal_mass_initial_temperatures=[25, 25] degC  thermal_mass_initial_temperatures_Cauer=[25, 25, 25] degC  junction_thermal_mass=0.1 J/K  Tvec_initial_Foster=[25, 25, 25, 25] degC  junction_temperature_specify=off  junction_temperature_priority=None  junction_temperature=25 degC  junction_temperature_nominal_specify=off  junction_temperature_nominal_unit=degC  junction_temperature_nominal_value=1
      settings: InternalSimscapePortConfiguration="{\"Bottom\":[{\"id\":\"n\",\"label\":\"-\",\"type\":\"foundation.electrical.electrical\"}],\"Left\":[{\"id\":\"G\",\"label\":\"G\",\"type\":\"input\"},{\"id\":\"H\",\"label\":\"\",\"type\":\"foundation.thermal.thermal\"}],\"Right\":[{\"id\":\"o\",\"label\":\"o\",\"type\":\"foundation.electrical.electrical\"}],\"Top\":[{\"id\":\"p\",\"label\":\"+\",\"type\":\"foundation.electrical.electrical\"}]}"
  Vb : PMIOPort  Side=Right
  Vc : PMIOPort  Port=2  Side=Right
  Va : PMIOPort  Port=3  Side=Right
  wires:
  PS-Simulink Converter8/1 -> Scope20/1
  PS-Simulink Converter9/1 -> Scope21/1
  Sa/Sa'/1 -> Simulink-PS Converter6/1
  Sb/Sb'/1 -> Simulink-PS Converter7/1
  Sc/Sc'/1 -> Simulink-PS Converter8/1
  connections:
  Voltage Sensor4/RConn1 -- PS-Simulink Converter9/LConn1
  Simulink-PS Converter8/RConn1 -- c/LConn1
  DC Voltage Source1/RConn1 -- Electrical Reference/LConn1 -- c/RConn2 -- a/RConn2 -- b/RConn2 -- Voltage Sensor4/RConn2 -- Voltage Sensor3/RConn2
  a/LConn3 -- Voltage Sensor4/LConn1 -- b/LConn3 -- Voltage Sensor3/LConn1 -- DC Voltage Source1/LConn1 -- c/LConn3
  Simulink-PS Converter6/RConn1 -- a/LConn1
  Voltage Sensor3/RConn1 -- PS-Simulink Converter8/LConn1
  b/LConn1 -- Simulink-PS Converter7/RConn1
  Va/RConn1 -- a/RConn1
  Vc/RConn1 -- c/RConn1
  Vb/RConn1 -- b/RConn1

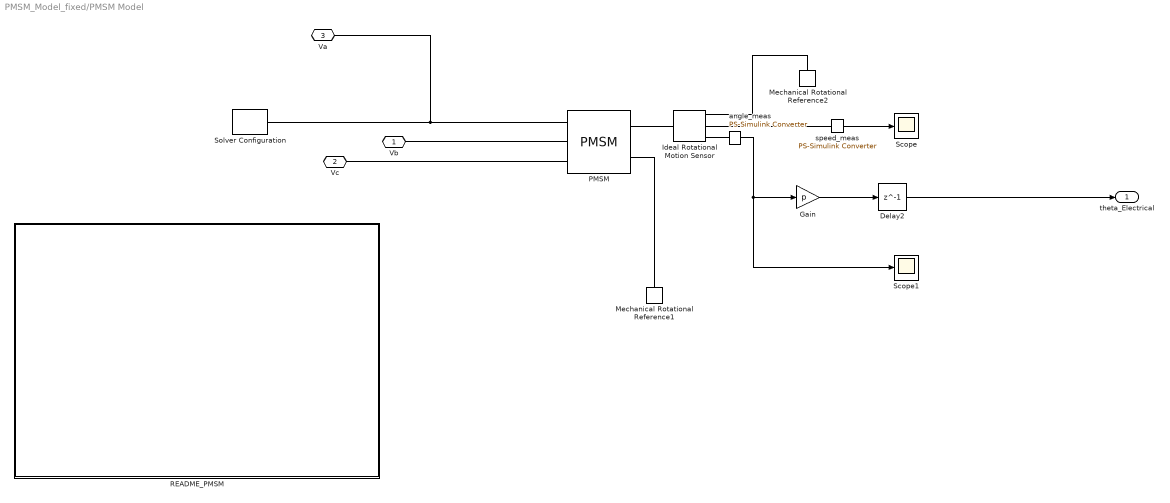
== system PMSM_Model_fixed/PMSM Model ==
  Delay2 : Delay  DelayLength=1  SampleTime=Ts_ctrl
  Gain : Gain  Gain=p
  Ideal Rotational Motion Sensor : fl_lib/Mechanical/Mechanical Sensors/Ideal Rotational Motion Sensor  reference=foundation.enum.MeasurementReference.difference  acceleration_port=false  velocity_port=true  position_port=true  wrap_angle=false  offset=0 rad
  Mechanical Rotational Reference1 : fl_lib/Mechanical/Rotational Elements/Mechanical Rotational Reference
  Mechanical Rotational Reference2 : fl_lib/Mechanical/Rotational Elements/Mechanical Rotational Reference
  PMSM : ee_lib/Electromechanical/Permanent Magnet/PMSM  port_option=ee.enum.threePhasePort.expanded  winding_type=ee.enum.statorconnection.wye  machine_param=ee.enum.pmsm.parameterization.constant  nPolePairs=p  pmflux_param=ee.enum.pmflux.fluxlinkage  pm_flux_linkage=0.01 Wb  torque_constant=0.18 N*m/A  back_emf_constant=0.18 V*s/rad  stator_param=ee.enum.statorparam.LdLqL0  Ld=1 mH  Lq=1 mH  idVec=[-200, 0, 200] A  iqVec=[-200, 0, 200] A  LdMatrix=0.0002 * ones(3, 3) H  LqMatrix=0.0002 * ones(3, 3) H  PmMatrix=0.1 * ones(3, 3) Wb  ktMatrix=0.18 * ones(3, 3) N*m/A  keMatrix=0.18 * ones(3, 3) V*s/rad  L0=0.00016 H  Ls=0.0002 H  Lm=-0.00002 H  Ms=0.00002 H  Rs=0.5 Ohm  zero_sequence=ee.enum.park.zerosequence.exclude  axes_param=ee.enum.rotorangle.daxis  loss_param=ee.enum.ironloss.none  losses_oc=[0, 0, 0] W  losses_sc=[0, 0, 0] W  f_losses=60 Hz  Isc_losses=95 A  J=0.0001 kg*m^2  lam=0.001 N*m/(rad/s)  i_d_specify=off  i_d_priority=None  i_d=0 A  i_d_nominal_specify=off  i_d_nominal_unit=A  i_d_nominal_value=1  i_q_specify=off  i_q_priority=None  i_q=0 A  i_q_nominal_specify=off  i_q_nominal_unit=A  i_q_nominal_value=1  torque_specify=off  torque_priority=None  torque=0 N*m  torque_nominal_specify=off  torque_nominal_unit=N*m  torque_nominal_value=1  angular_velocity_specify=off  angular_velocity_priority=High  angular_velocity=0 rpm  angular_velocity_nominal_specify=off  angular_velocity_nominal_unit=rpm  angular_velocity_nominal_value=1  angular_position_specify=off  angular_position_priority=High  angular_position=0 deg  angular_position_nominal_specify=off  angular_position_nominal_unit=deg  angular_position_nominal_value=1  alpha=3.93e-3 1/K  alpha_flux=-0.001 1/K  Tmeas=298.15 K  stator_thermal_mass=100 J/K  rotor_thermal_mass=200 J/K  Rm_percent_rotor=90  Rd_percent_rotor=30  temperatureA_specify=off  temperatureA_priority=High  temperatureA=25 degC  temperatureA_nominal_specify=off  temperatureA_nominal_unit=degC  temperatureA_nominal_value=1  temperatureB_specify=off  temperatureB_priority=High  temperatureB=25 degC  temperatureB_nominal_specify=off  temperatureB_nominal_unit=degC  temperatureB_nominal_value=1  temperatureC_specify=off  temperatureC_priority=High  temperatureC=25 degC  temperatureC_nominal_specify=off  temperatureC_nominal_unit=degC  temperatureC_nominal_value=1  temperatureR_specify=off  temperatureR_priority=High  temperatureR=25 degC  temperatureR_nominal_specify=off  temperatureR_nominal_unit=degC  temperatureR_nominal_value=1
      settings: LogSimulationData=on  InternalSimscapePortConfiguration="{\"Bottom\":[],\"Left\":[{\"id\":\"a\",\"label\":\"a\",\"type\":\"foundation.electrical.electrical\"},{\"id\":\"b\",\"label\":\"b\",\"type\":\"foundation.electrical.electrical\"},{\"id\":\"c\",\"label\":\"c\",\"type\":\"foundation.electrical.electrical\"}],\"Right\":[{\"id\":\"R\",\"label\":\"R\",\"type\":\"foundation.mechanical.rotational.rotational\"},{\"id\":\"C\",\"label\":\"C\",\"type\":\"foundation.mechanical.rotational.rotational\"}],\"Top\":[]}"
  README_PMSM : Subsystem  InitFcn=docblock('save_document',gcb);  mask(DocBlock){ECoderFlag=, DocumentType=Text}
      mask prompts: ECoderFlag "Simulink:masks:DocBlockEmbeddedCoderFlagLabel_MP"; DocumentType "Simulink:masks:DocBlockDocTypeLabel_MP"
      mask help:
      | PMSM 本体 + 位置反馈
      |
      | 【物理端口】注意块上从左到右的顺序是 Vb / Vc / Va，不是 a/b/c：
      |     Va (LConn3) -> PMSM 的 a 相        Vb (LConn1) -> b 相
      |     Vc (LConn2) -> c 相
      |   接线时请按端口名而不是按位置，避免相序接错。
      |
      | 【输出】
      |     theta_Electrical = p * theta_mech  [rad]，Park / 反 Park 共用
      |
      | 【内部】
      |     PMSM：Ld = Lq = 1 mH（表贴式）、psi_f = 0.01 Wb、Rs = 0.5 ohm、
      |           p = 6、J = 1e-4 kg*m^2、lam = 1e-3 N*m/(rad/s)
      |     Ideal Rotational Motion Sensor：wrap_angle = off（角度连续累加）
      |     角度链：Gain(p) -> Delay2(Ts_ctrl) -> theta_Electrical
      |     Solver Configuration：本电气网络的求解器入口
      |     speed_meas / angle_meas：转速与角度取出给内部 Scope
      |
      | 【为什么没有开环起动（I/F）】
      |   该电机 J = 1e-4、iq = 1 A 时机械角加速度约 900 rad/s^2，
      |   而常见的开环斜坡只有 10 Hz 电气量级，转子会立刻冲出同步区失步。
      |   带真实位置传感器时，直接闭环起动才是正确做法。
      |   如需练习 I/F 起动，需把斜坡斜率提到与加速度匹配的数量级，并做切换点平滑。
      settings: DeleteFcn=docblock('close_document',gcb);  PreSaveFcn=docblock('save_document',gcb);  OpenFcn=docblock('edit_document',gcb);
      settings: LibrarySourceBlock=|
      | simulink/Model-Wide
      | Utilities/DocBlock
      mask TypeOptions DocumentType: Simulink:masks:Text | Simulink:masks:RTF | Simulink:masks:HTML
      mask Display:
      | plot([.8 0 0 1 1 .8 .8 1],[1 1 0 0 .8 1 .8 .8]);
      | text(.5,.6,'DOC','horizontalalignment','center');
      | text(.95,.05,get_param(gcb,'DocumentType'),'verticalalignment','bottom','horizontalalignment','right');
  Scope : Scope
  Scope1 : Scope
  Solver Configuration : nesl_utility/Solver Configuration  PhysicalDomain=network_engine_domain  SubClassName=solver  LeftPortType=input  RightPortType=generic  Tones=[]  Harmonics=[]  SimulateNoise=off  Profile=off  UseLocalSampling=off  EnableSwitchedLinearOptims=on  FrequencyDomain=off  UseCCode=off  RelTol=0.001  AbsTol=0.001  MinStep=1e-09  ToWorkspace=off  RevertToSquareIcSolve=off  NumHomotopyIterations=100  PhasorMode=off  PhasorModeNumHarmonics=1  ConsistencySolver=NEWTON_XTOL_AFTER_FTOL  IndexReductionMethod=DerivativeReplacement  DoDC=off  ResidualTolerance=1e-09  ConsistencyTolSource=GLOBAL  ConsistencyAbsTol=0.001  ConsistencyRelTol=0.001  ConsistencyTolFactor=1e-3  UseLocalSolver=off  LocalSolverChoice=NE_BACKWARD_EULER_ADVANCER  ResolveIndetEquations=on  FunctionEvalNumThread=1  LocalSolverSampleTime=0.001  DoFixedCost=off  MaxNonlinIter=3  MaxModeIter=2  ComputeImpulses=off  ImpulseIterations=2  LinearAlgebra=auto  LinearAlgebraNumThread=0  EquationFormulation=NE_TIME_EF  DelaysMemoryBudget=1024  AutomaticFiltering=on  FilteringTimeConstant=0.001  PartitionStorageMethod=AS_NEEDED  PartitionMemoryBudget=1024  PartitionMethod=ROBUST
  angle_meas : nesl_utility/PS-Simulink Converter  PhysicalDomain=network_engine_domain  SubClassName=ps_output  LeftPortType=input  RightPortType=output  PseudoPeriodic=off  Frequencies=[]  VectorFormat=inherit  Unit=rad  AffineConversion=off
  speed_meas : nesl_utility/PS-Simulink Converter  PhysicalDomain=network_engine_domain  SubClassName=ps_output  LeftPortType=input  RightPortType=output  PseudoPeriodic=off  Frequencies=[]  VectorFormat=inherit  Unit=rad/s  AffineConversion=off
  Vb : PMIOPort  Side=Left
  Vc : PMIOPort  Port=2  Side=Left
  Va : PMIOPort  Port=3  Side=Left
  theta_Electrical : Outport
  wires:
  speed_meas/1 -> Scope/1
  angle_meas/1 -> Gain/1, Scope1/1
  Gain/1 -> Delay2/1
  Delay2/1 -> theta_Electrical/1
  connections:
  PMSM/RConn1 -- Ideal Rotational Motion Sensor/LConn1
  Ideal Rotational Motion Sensor/RConn2 -- speed_meas/LConn1
  PMSM/RConn2 -- Mechanical Rotational Reference1/LConn1
  Ideal Rotational Motion Sensor/RConn3 -- angle_meas/LConn1
  Solver Configuration/RConn1 -- Va/RConn1 -- PMSM/LConn1
  Ideal Rotational Motion Sensor/RConn1 -- Mechanical Rotational Reference2/LConn1
  PMSM/LConn3 -- Vc/RConn1
  Vb/RConn1 -- PMSM/LConn2

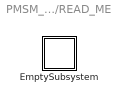
== system PMSM_Model_fixed/READ_ME ==
  EmptySubsystem : Subsystem

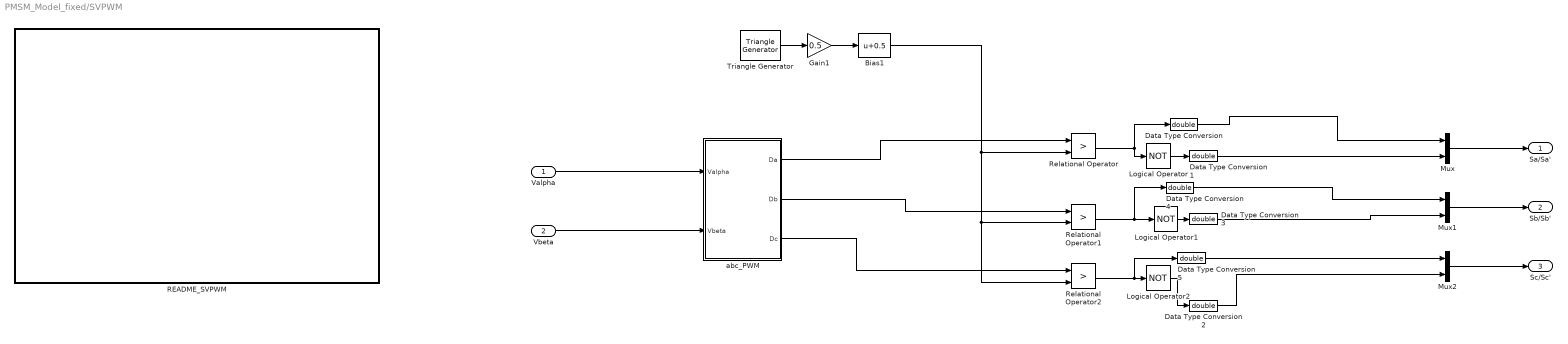
== system PMSM_Model_fixed/SVPWM ==
  Valpha : Inport
  Vbeta : Inport  Port=2
  Bias1 : Bias  Bias=0.5  SaturateOnIntegerOverflow=off
  Data Type Conversion{,1..5} (6 alike) : DataTypeConversion  OutDataTypeStr=double  SaturateOnIntegerOverflow=off  RndMeth=Floor
  Gain1 : Gain  Gain=0.5
  Logical Operator : Logic  Operator=NOT  AllPortsSameDT=off  OutDataTypeStr=boolean
  Logical Operator1 : Logic  Operator=NOT  AllPortsSameDT=off  OutDataTypeStr=boolean
  Logical Operator2 : Logic  Operator=NOT  AllPortsSameDT=off  OutDataTypeStr=boolean
  Mux : Mux  Inputs=2
  Mux1 : Mux  Inputs=2
  Mux2 : Mux  Inputs=2
  README_SVPWM : Subsystem  InitFcn=docblock('save_document',gcb);  mask(DocBlock){ECoderFlag=, DocumentType=Text}
      mask prompts: ECoderFlag "Simulink:masks:DocBlockEmbeddedCoderFlagLabel_MP"; DocumentType "Simulink:masks:DocBlockDocTypeLabel_MP"
      mask help:
      | 空间矢量调制 + 载波比较 + 互补门极生成
      |
      | 【接口】输入 Valpha / Vbeta；输出 Sa/Sa'、Sb/Sb'、Sc/Sc'（每路 2 元素门极向量）
      |
      | 【内部】
      |   abc_PWM            -> Da / Db / Dc（0~1 占空比）
      |   Triangle Generator -> Freq = fsw = 10 kHz，输出 -1 ~ +1 双极性三角波
      |   Gain1 = 0.5、Bias1 = +0.5  -> 抬成 0 ~ 1 单极性载波
      |   Relational Operator (Da > carrier) + NOT + Mux -> 互补门极对
      |   Scope Da&Db&Dc     -> 三相占空比
      |
      | 【重要约定：Ts_norm = 1】
      |   abc_PWM 里 T1/T2 的公式按 Ts = 1 计算，因此 Da/Db/Dc 直接就是占空比，
      |   可以直接和 0~1 的载波比较。若把 Ts 改成 1e-4，占空比会缩小 10000 倍。
      |
      | 【abc_PWM 的三个函数】
      |   sector_calc   扇区号 1..6 = floor(angle/(pi/3)) + 1
      |   T1T2_calc     T1 = sqrt(3)*Ts*|V|/Vdc*sin(60-theta')，T2 = ...*sin(theta')
      |   duty_to_abc   七段式占空比表（已用 min/max 共模注入法交叉校验）
      settings: DeleteFcn=docblock('close_document',gcb);  PreSaveFcn=docblock('save_document',gcb);  OpenFcn=docblock('edit_document',gcb);
      settings: LibrarySourceBlock=|
      | simulink/Model-Wide
      | Utilities/DocBlock
      mask TypeOptions DocumentType: Simulink:masks:Text | Simulink:masks:RTF | Simulink:masks:HTML
      mask Display:
      | plot([.8 0 0 1 1 .8 .8 1],[1 1 0 0 .8 1 .8 .8]);
      | text(.5,.6,'DOC','horizontalalignment','center');
      | text(.95,.05,get_param(gcb,'DocumentType'),'verticalalignment','bottom','horizontalalignment','right');
  Relational Operator : RelationalOperator  Operator=>  OutDataTypeStr=boolean  RndMeth=Simplest  InputSameDT=off
  Relational Operator1 : RelationalOperator  Operator=>  OutDataTypeStr=boolean  RndMeth=Simplest  InputSameDT=off
  Relational Operator2 : RelationalOperator  Operator=>  OutDataTypeStr=boolean  RndMeth=Simplest  InputSameDT=off
  Triangle Generator : spsTriangleGeneratorLib/Triangle Generator  Freq=fsw  Phase=0  Ts=1e-6
  abc_PWM : Subsystem
  Sa/Sa' : Outport
  Sb/Sb' : Outport  Port=2
  Sc/Sc' : Outport  Port=3
  wires:
  Triangle Generator/1 -> Gain1/1
  Data Type Conversion5/1 -> Mux2/1
  Mux2/1 -> Sc/Sc'/1
  Bias1/1 -> Relational Operator/2, Relational Operator1/2, Relational Operator2/2
  Relational Operator/1 -> Data Type Conversion/1, Logical Operator/1
  Valpha/1 -> abc_PWM/1(Valpha)
  Relational Operator1/1 -> Data Type Conversion4/1, Logical Operator1/1
  Logical Operator2/1 -> Data Type Conversion2/1
  Logical Operator/1 -> Data Type Conversion1/1
  Gain1/1 -> Bias1/1
  Data Type Conversion/1 -> Mux/1
  Data Type Conversion4/1 -> Mux1/1
  abc_PWM/1(Da) -> Relational Operator/1
  Relational Operator2/1 -> Data Type Conversion5/1, Logical Operator2/1
  Data Type Conversion2/1 -> Mux2/2
  Data Type Conversion1/1 -> Mux/2
  Mux/1 -> Sa/Sa'/1
  abc_PWM/2(Db) -> Relational Operator1/1
  Data Type Conversion3/1 -> Mux1/2
  Logical Operator1/1 -> Data Type Conversion3/1
  abc_PWM/3(Dc) -> Relational Operator2/1
  Mux1/1 -> Sb/Sb'/1
  Vbeta/1 -> abc_PWM/2(Vbeta)

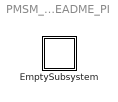
== system PMSM_Model_fixed/Current_PI/README_PI ==
  EmptySubsystem : Subsystem

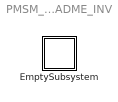
== system PMSM_Model_fixed/Inverter/README_INV ==
  EmptySubsystem : Subsystem

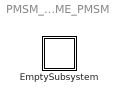
== system PMSM_Model_fixed/PMSM Model/README_PMSM ==
  EmptySubsystem : Subsystem

== system PMSM_Model_fixed/READ_ME/EmptySubsystem ==

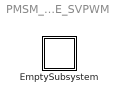
== system PMSM_Model_fixed/SVPWM/README_SVPWM ==
  EmptySubsystem : Subsystem

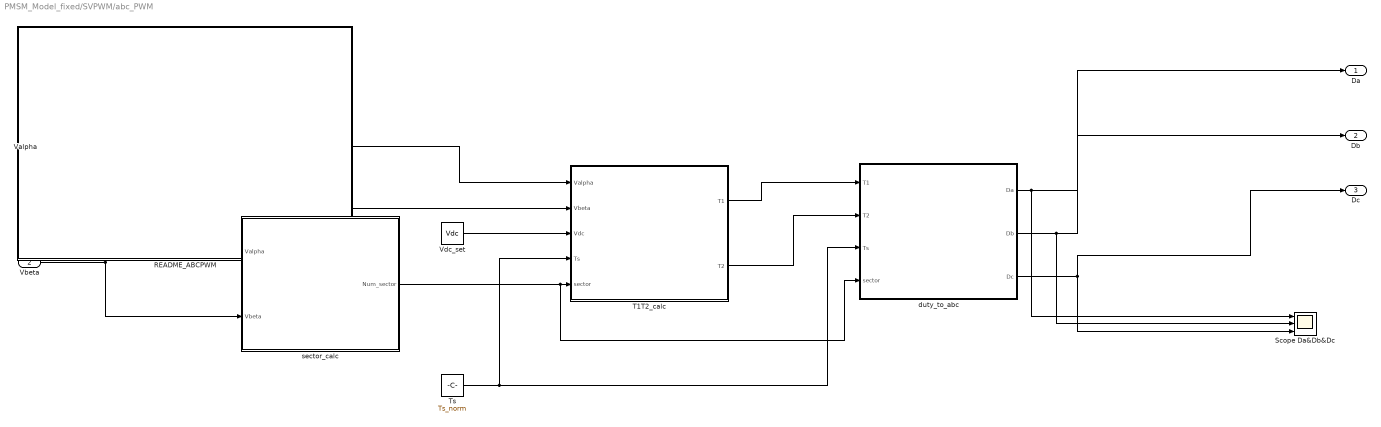
== system PMSM_Model_fixed/SVPWM/abc_PWM ==
  Valpha : Inport
  Vbeta : Inport  Port=2
  README_ABCPWM : Subsystem  InitFcn=docblock('save_document',gcb);  mask(DocBlock){ECoderFlag=, DocumentType=Text}
      mask prompts: ECoderFlag "Simulink:masks:DocBlockEmbeddedCoderFlagLabel_MP"; DocumentType "Simulink:masks:DocBlockDocTypeLabel_MP"
      mask help:
      | SVPWM 核心计算：Valpha / Vbeta -> Da / Db / Dc
      |
      |   sector_calc  ->  T1T2_calc  ->  duty_to_abc
      |
      |   Vdc = 100（模型工作区变量）
      |   Ts  = 1  （归一化，令 Da/Db/Dc 直接就是占空比；详见 SVPWM 的说明）
      settings: DeleteFcn=docblock('close_document',gcb);  PreSaveFcn=docblock('save_document',gcb);  OpenFcn=docblock('edit_document',gcb);
      settings: LibrarySourceBlock=|
      | simulink/Model-Wide
      | Utilities/DocBlock
      mask TypeOptions DocumentType: Simulink:masks:Text | Simulink:masks:RTF | Simulink:masks:HTML
      mask Display:
      | plot([.8 0 0 1 1 .8 .8 1],[1 1 0 0 .8 1 .8 .8]);
      | text(.5,.6,'DOC','horizontalalignment','center');
      | text(.95,.05,get_param(gcb,'DocumentType'),'verticalalignment','bottom','horizontalalignment','right');
  Scope Da&Db&Dc : Scope  NumInputPorts=3
  T1T2_calc : MATLAB Function  TreatAsAtomicUnit=on
  Ts : Constant  Value=Ts_norm
  Vdc_set : Constant  Value=Vdc
  duty_to_abc : MATLAB Function  TreatAsAtomicUnit=on
  sector_calc : MATLAB Function  TreatAsAtomicUnit=on
  Da : Outport
  Db : Outport  Port=2
  Dc : Outport  Port=3
  wires:
  Ts/1 -> duty_to_abc/3(Ts), T1T2_calc/4(Ts)
  duty_to_abc/2(Db) -> Db/1, Scope Da&Db&Dc/2
  duty_to_abc/3(Dc) -> Dc/1, Scope Da&Db&Dc/3
  sector_calc/1(Num_sector) -> duty_to_abc/4(sector), T1T2_calc/5(sector)
  T1T2_calc/1(T1) -> duty_to_abc/1(T1)
  T1T2_calc/2(T2) -> duty_to_abc/2(T2)
  Vdc_set/1 -> T1T2_calc/3(Vdc)
  duty_to_abc/1(Da) -> Scope Da&Db&Dc/1, Da/1
  Vbeta/1 -> sector_calc/2(Vbeta), T1T2_calc/2(Vbeta)
  Valpha/1 -> sector_calc/1(Valpha), T1T2_calc/1(Valpha)

== system PMSM_Model_fixed/Current_PI/README_PI/EmptySubsystem ==

== system PMSM_Model_fixed/Inverter/README_INV/EmptySubsystem ==

== system PMSM_Model_fixed/PMSM Model/README_PMSM/EmptySubsystem ==

== system PMSM_Model_fixed/SVPWM/README_SVPWM/EmptySubsystem ==

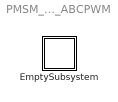
== system PMSM_Model_fixed/SVPWM/abc_PWM/README_ABCPWM ==
  EmptySubsystem : Subsystem

== system PMSM_Model_fixed/SVPWM/abc_PWM/README_ABCPWM/EmptySubsystem ==

== matlab function PMSM_Model_fixed/Park Trans ==
  settings: updateMethod=DISCRETE  sampleTime=1e-4
  data: ialpha input; id output; ibeta input; theta_Electrical input; iq output
function [id, iq] = park(ialpha, ibeta, theta_Electrical)
    % Park 变换：两相静止 -> 两相旋转
    id = ialpha * cos(theta_Electrical) + ibeta * sin(theta_Electrical);
    iq = -ialpha * sin(theta_Electrical) + ibeta * cos(theta_Electrical);
end

== matlab function PMSM_Model_fixed/Clarke Trans ==
  settings: updateMethod=DISCRETE  sampleTime=1e-4
  data: ia input; i_alpha output; ib input; i_beta output
function [i_alpha,i_beta] = fcn(ia,ib)

i_alpha = ia;
i_beta = (1/sqrt(3))*(ia + 2*ib);

== matlab function PMSM_Model_fixed/Current_PI/Vd_func ==
  settings: updateMethod=DISCRETE  sampleTime=1e-4
  data: Kp input; Ki input; error input; Vd output
function Vd = fcn(Kp,Ki,error)
% Discrete PI current controller, one step per Ts = 1e-4 s.
% The original code began with "integral = 0" on every call, so the
% integral term never accumulated and the loop had no integral action.
    persistent integral
    Ts    = 1e-4;
    limit = 57;      % Vdc/sqrt(3) = 100/sqrt(3): linear SVPWM limit
    if isempty(integral)
        integral = 0;
    end
    integral = integral + error*Ts;
    if Ki ~= 0
        if Ki*integral >  limit
            integral =  limit/Ki;
        end
        if Ki*integral < -limit
            integral = -limit/Ki;
        end
    end
    Vd = Kp*error + Ki*integral;
    if Vd >  limit
        Vd =  limit;
    end
    if Vd < -limit
        Vd = -limit;
    end
end

== matlab function PMSM_Model_fixed/Current_PI/Vq_func ==
  settings: updateMethod=DISCRETE  sampleTime=1e-4
  data: Kp input; Ki input; error input; Vq output
function Vq = fcn(Kp,Ki,error)
% Discrete PI current controller, one step per Ts = 1e-4 s.
% The original code began with "integral = 0" on every call, so the
% integral term never accumulated and the loop had no integral action.
    persistent integral
    Ts    = 1e-4;
    limit = 57;      % Vdc/sqrt(3) = 100/sqrt(3): linear SVPWM limit
    if isempty(integral)
        integral = 0;
    end
    integral = integral + error*Ts;
    if Ki ~= 0
        if Ki*integral >  limit
            integral =  limit/Ki;
        end
        if Ki*integral < -limit
            integral = -limit/Ki;
        end
    end
    Vq = Kp*error + Ki*integral;
    if Vq >  limit
        Vq =  limit;
    end
    if Vq < -limit
        Vq = -limit;
    end
end

== matlab function PMSM_Model_fixed/INV_Park ==
  settings: updateMethod=DISCRETE  sampleTime=1e-4
  data: Vd input; Valpha output; Vq input; theta_Electrical input; Vbeta output
function [Valpha, Vbeta] = inv_park(Vd, Vq, theta_Electrical)
    Valpha = Vd * cos(theta_Electrical) - Vq * sin(theta_Electrical);
    Vbeta  = Vd * sin(theta_Electrical) + Vq * cos(theta_Electrical);
end

== matlab function PMSM_Model_fixed/SVPWM/abc_PWM/sector_calc ==
  settings: updateMethod=DISCRETE  sampleTime=1e-4
  data: Valpha input; Num_sector output; Vbeta input
function Num_sector = SVPWM_Sector(Valpha,Vbeta)
% Sector index 1..6, counter-clockwise starting on the alpha axis.
% The original floor((pi*angel)/3)+1 was a typo for floor(angel/(pi/3))+1
% and selected the wrong sector over most of the circle.
    angel = atan2(Vbeta,Valpha);
    if angel < 0
        angel = angel + 2*pi;
    end
    Num_sector = floor(angel/(pi/3)) + 1;
    Num_sector = max(1, min(6, Num_sector));
end

== matlab function PMSM_Model_fixed/SVPWM/abc_PWM/T1T2_calc ==
  settings: updateMethod=DISCRETE  sampleTime=1e-4
  data: Valpha input; T1 output; Vbeta input; Vdc input; Ts input; sector input; T2 output
function [T1, T2] = svpwm_time(Valpha, Vbeta, Vdc, Ts, sector)
    % 目标矢量幅值
    Vmag = sqrt(Valpha^2 + Vbeta^2);
    
    % 目标矢量角度
    angle = atan2(Vbeta, Valpha);
    if angle < 0
        angle = angle + 2*pi;
    end
    
    % 相对于扇区起始边的角度
    theta_prime = angle - (sector - 1) * pi/3;
    
    % 计算 T1, T2
    T1 = sqrt(3) * Ts * Vmag / Vdc * sin(pi/3 - theta_prime);
    T2 = sqrt(3) * Ts * Vmag / Vdc * sin(theta_prime);
end

== matlab function PMSM_Model_fixed/SVPWM/abc_PWM/duty_to_abc ==
  settings: updateMethod=DISCRETE  sampleTime=1e-4
  data: T1 input; Da output; T2 input; Ts input; sector input; Db output; Dc output
function [Da, Db, Dc] = svpwm_duty(T1, T2, Ts, sector)
% Symmetric 7-segment SVPWM duty cycles for phases a, b and c.
% T1 is the on-time of the sector-start vector, T2 that of the next one.
% Ts is the PWM period; this model feeds Ts = 1, so Da/Db/Dc are duty
% ratios that are compared against a 0..1 carrier.
    Ta = (Ts - T1 - T2)/2;      % half of the zero-vector time
    Da = 0; Db = 0; Dc = 0;
    switch round(sector)
        case 1
            Da = Ta + T1 + T2;  Db = Ta + T2;        Dc = Ta;
        case 2
            Da = Ta + T1;       Db = Ta + T1 + T2;   Dc = Ta;
        case 3
            Da = Ta;            Db = Ta + T1 + T2;   Dc = Ta + T2;
        case 4
            Da = Ta;            Db = Ta + T1;        Dc = Ta + T1 + T2;
        case 5
            Da = Ta + T2;       Db = Ta;             Dc = Ta + T1 + T2;
        case 6
            Da = Ta + T1 + T2;  Db = Ta;             Dc = Ta + T1;
    end
    Da = min(max(Da,0),Ts);
    Db = min(max(Db,0),Ts);
    Dc = min(max(Dc,0),Ts);
end
